simulink model "Copy_of_towing_project1"  (Simulink 10.1)
settings: Solver=ode4  StartTime=0.0  StopTime=200  FixedStep=1  RelTol=1e-3  EnableMultiTasking=on
PreLoadFcn:
  | load('Initialization_data.mat');
values from neighbouring files (symbols this model uses):
  D1 = [MM(1,1)/100, 0, 0; 0, MM(2,2)/40, 0; 0, 0, MM(3,3)/20]    [temp_code.m]
  M1 = diag([6.25e5, 6.25e5, 6.25e5*7.5^2])    [temp_code.m]
  Ma1 = [7.58e4, 0, 0; 0, 3.69e5 -1.4e5; 0, -1.4e5, 8.77e6]    [temp_code.m]
undefined symbols (not defined in the file or in its folder): magnitude
libraries: simulink_extras x4, simulink x4
settings Model: Creator=Lither  LastModifiedBy=Administrator
settings DataIOCC: LimitDataPoints=on
settings OptimizationCC: ExpressionDepthLimit=2147483647
settings DebuggingCC: FcnCallInpInsideContextMsg=warning  StateNameClashWarn=warning
settings ConfigComp: CovSFcnEnable=off

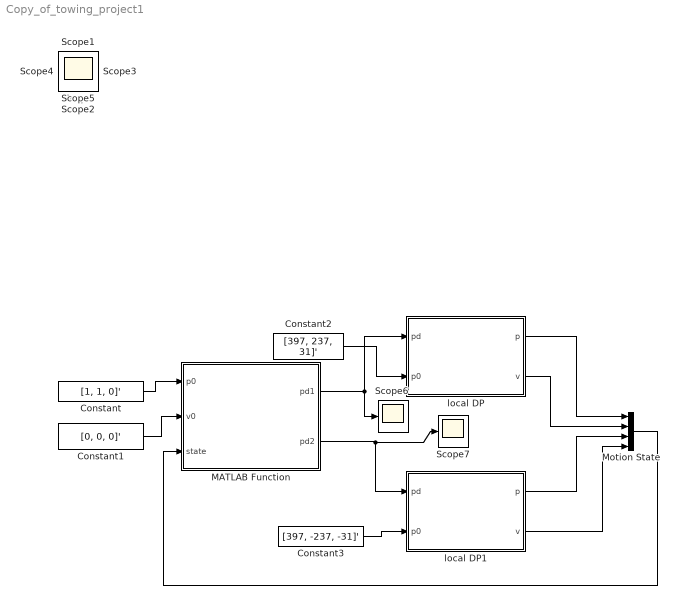
== system Copy_of_towing_project1 ==
  Constant : Constant  Value=[1, 1, 0]'
  Constant1 : Constant  Value=[0, 0, 0]'
  Constant2 : Constant  Value=[397, 237, 31]'
  Constant3 : Constant  Value=[397, -237, -31]'
  MATLAB Function : MATLAB Function  TreatAsAtomicUnit=on
  Motion State : Mux
  Scope{,1..7} (8 alike) : Scope
  local DP : Subsystem
  local DP1 : Subsystem
  wires:
  Constant/1 -> MATLAB Function/1(p0)
  Constant1/1 -> MATLAB Function/2(v0)
  MATLAB Function/1(pd1) -> local DP/1(pd), Scope6/1
  MATLAB Function/2(pd2) -> Scope7/1, local DP1/1(pd)
  Constant2/1 -> local DP/2(p0)
  Constant3/1 -> local DP1/2(p0)
  local DP/1(p) -> Motion State/1
  local DP/2(v) -> Motion State/2
  local DP1/1(p) -> Motion State/3
  local DP1/2(v) -> Motion State/4
  Motion State/1 -> MATLAB Function/3(state)

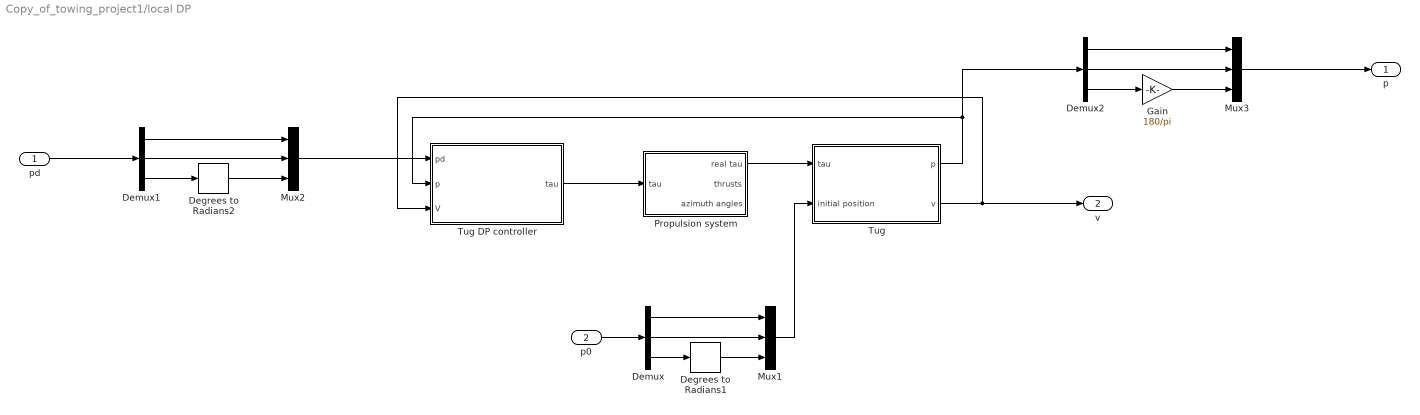
== system Copy_of_towing_project1/local DP ==
  pd : Inport
  p0 : Inport  Port=2
  Degrees to Radians1 : simulink_extras/Transformations/Degrees to Radians
  Degrees to Radians2 : simulink_extras/Transformations/Degrees to Radians
  Demux : Demux  Outputs=3
  Demux1 : Demux  Outputs=3
  Demux2 : Demux  Outputs=3
  Gain : Gain  Gain=180/pi
  Mux1 : Mux  Inputs=3
  Mux2 : Mux  Inputs=3
  Mux3 : Mux  Inputs=3
  Propulsion system : Subsystem  mask{f0=[1;1;1], a0=[50;60;70], u0=[1; 1; 1], wa=on}
      mask prompts: f0 "Initial values of thrusts"; a0 "Initial values of azimuth angles"; u0 "Thruster utilization"; wa "Show animation of thrust and azimuth angle"
  Tug : Subsystem  mask{wv=on}
      mask prompts: wv "Display animation of the vessel's motion"
  Tug DP controller : Subsystem  mask(Nonlinear DP Controller){Kp=diag([0.0028, 0.004, 0.0031]), Kd=diag([0.0573, 0.0716, 0.025]), Ki=diag([0.0028, 0.004, 0.0031])*0.01, WFF_gain=0}
      mask prompts: Kp "Proportional Gain Matrix: Kp"; Kd "Derivative Gain Matrix: Kd"; Ki "Integral Gain Matrix: Ki"; WFF_gain "Wave feedforward Gain"
      mask help: PID controller for Set-Point Reulation in Surge, Sway and Yaw
      mask Help:
      | The nonlinear  PID controller uses the rotation matrix in yaw for proper scaling of the surge, sway and yaw gains as a function of the yaw angle.
      | INPUTS: (1) eta_ref, (2) eta, (3) nu. OUPUTS: (1) tau.
      mask Display: disp('PID controller')
  p : Outport
  v : Outport  Port=2
  wires:
  Tug/2(v) -> v/1, Tug DP controller/3(V)
  Demux/2 -> Mux1/2
  Tug DP controller/1(tau) -> Propulsion system/1(tau)
  Demux1/2 -> Mux2/2
  Mux2/1 -> Tug DP controller/1(pd)
  Demux1/1 -> Mux2/1
  Degrees to Radians2/1 -> Mux2/3
  Demux1/3 -> Degrees to Radians2/1
  pd/1 -> Demux1/1
  Demux/1 -> Mux1/1
  Degrees to Radians1/1 -> Mux1/3
  Demux/3 -> Degrees to Radians1/1
  Propulsion system/1(real tau) -> Tug/1(tau)
  Mux1/1 -> Tug/2(initial position)
  p0/1 -> Demux/1
  Demux2/2 -> Mux3/2
  Tug/1(p) -> Demux2/1, Tug DP controller/2(p)
  Mux3/1 -> p/1
  Demux2/3 -> Gain/1
  Gain/1 -> Mux3/3
  Demux2/1 -> Mux3/1

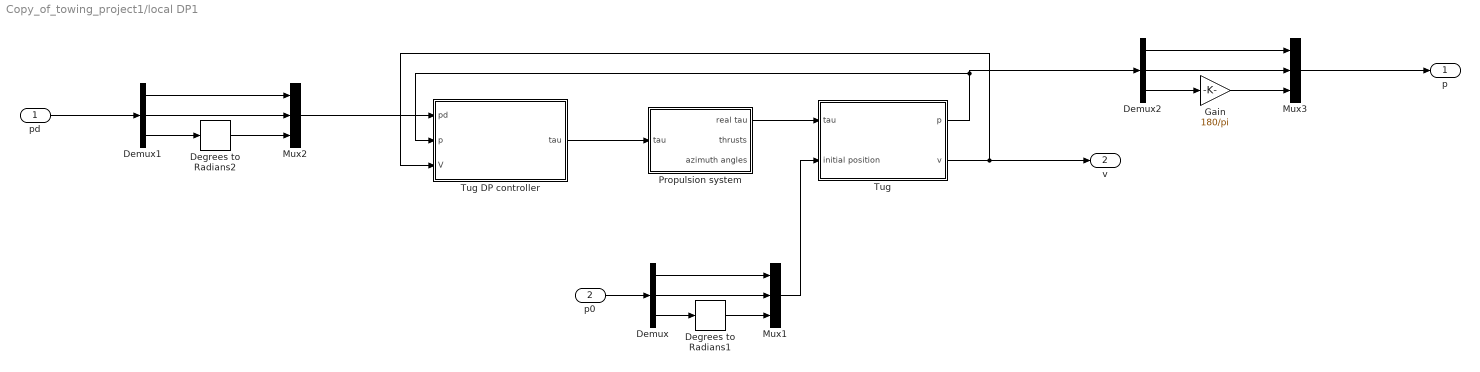
== system Copy_of_towing_project1/local DP1 ==
  pd : Inport
  p0 : Inport  Port=2
  Degrees to Radians1 : simulink_extras/Transformations/Degrees to Radians
  Degrees to Radians2 : simulink_extras/Transformations/Degrees to Radians
  Demux : Demux  Outputs=3
  Demux1 : Demux  Outputs=3
  Demux2 : Demux  Outputs=3
  Gain : Gain  Gain=180/pi
  Mux1 : Mux  Inputs=3
  Mux2 : Mux  Inputs=3
  Mux3 : Mux  Inputs=3
  Propulsion system : Subsystem  mask{f0=[1;1;1], a0=[50;60;70], u0=[1; 1; 1], wa=on}
      mask prompts: f0 "Initial values of thrusts"; a0 "Initial values of azimuth angles"; u0 "Thruster utilization"; wa "Show animation of thrust and azimuth angle"
  Tug : Subsystem  mask{wv=on}
      mask prompts: wv "Display animation of the vessel's motion"
  Tug DP controller : Subsystem  mask(Nonlinear DP Controller){Kp=diag([0.0028, 0.004, 0.0031]), Kd=diag([0.0573, 0.0716, 0.025]), Ki=diag([0.0028, 0.004, 0.0031])*0.01, WFF_gain=0}
      mask prompts: Kp "Proportional Gain Matrix: Kp"; Kd "Derivative Gain Matrix: Kd"; Ki "Integral Gain Matrix: Ki"; WFF_gain "Wave feedforward Gain"
      mask help: PID controller for Set-Point Reulation in Surge, Sway and Yaw
      mask Help:
      | The nonlinear  PID controller uses the rotation matrix in yaw for proper scaling of the surge, sway and yaw gains as a function of the yaw angle.
      | INPUTS: (1) eta_ref, (2) eta, (3) nu. OUPUTS: (1) tau.
      mask Display: disp('PID controller')
  p : Outport
  v : Outport  Port=2
  wires:
  Tug/2(v) -> v/1, Tug DP controller/3(V)
  Demux/2 -> Mux1/2
  Tug DP controller/1(tau) -> Propulsion system/1(tau)
  Demux1/2 -> Mux2/2
  Mux2/1 -> Tug DP controller/1(pd)
  Demux1/1 -> Mux2/1
  Degrees to Radians2/1 -> Mux2/3
  Demux1/3 -> Degrees to Radians2/1
  pd/1 -> Demux1/1
  Demux/1 -> Mux1/1
  Degrees to Radians1/1 -> Mux1/3
  Demux/3 -> Degrees to Radians1/1
  Propulsion system/1(real tau) -> Tug/1(tau)
  Mux1/1 -> Tug/2(initial position)
  p0/1 -> Demux/1
  Mux3/1 -> p/1
  Tug/1(p) -> Demux2/1, Tug DP controller/2(p)
  Demux2/3 -> Gain/1
  Demux2/2 -> Mux3/2
  Gain/1 -> Mux3/3
  Demux2/1 -> Mux3/1

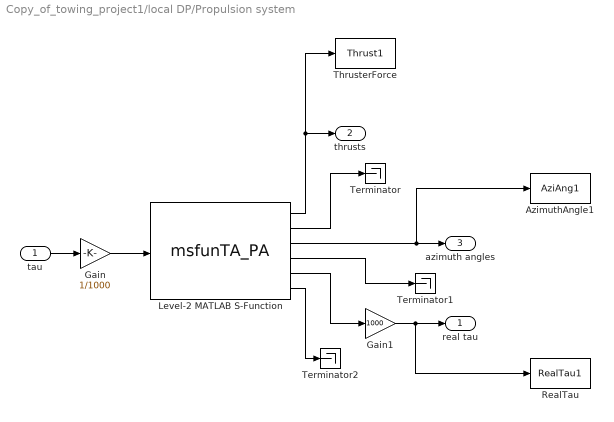
== system Copy_of_towing_project1/local DP/Propulsion system ==
  tau : Inport
  AzimuthAngle1 : ToWorkspace  VariableName=AziAng1  SampleTime=-1
  Gain : Gain  Gain=1/1000
  Gain1 : Gain  Gain=1000
  Level-2 MATLAB S-Function : M-S-Function  FunctionName=msfunTA_PA  Parameters=f0,a0,wa
  RealTau : ToWorkspace  VariableName=RealTau1  SampleTime=-1
  Terminator : Terminator
  Terminator1 : Terminator
  Terminator2 : Terminator
  ThrusterForce : ToWorkspace  VariableName=Thrust1  SampleTime=-1
  real tau : Outport
  thrusts : Outport  Port=2
  azimuth angles : Outport  Port=3
  wires:
  tau/1 -> Gain/1
  Level-2 MATLAB S-Function/2 -> Terminator/1
  Level-2 MATLAB S-Function/3 -> AzimuthAngle1/1, azimuth angles/1
  Level-2 MATLAB S-Function/4 -> Terminator1/1
  Level-2 MATLAB S-Function/5 -> Gain1/1
  Level-2 MATLAB S-Function/6 -> Terminator2/1
  Level-2 MATLAB S-Function/1 -> ThrusterForce/1, thrusts/1
  Gain/1 -> Level-2 MATLAB S-Function/1
  Gain1/1 -> RealTau/1, real tau/1

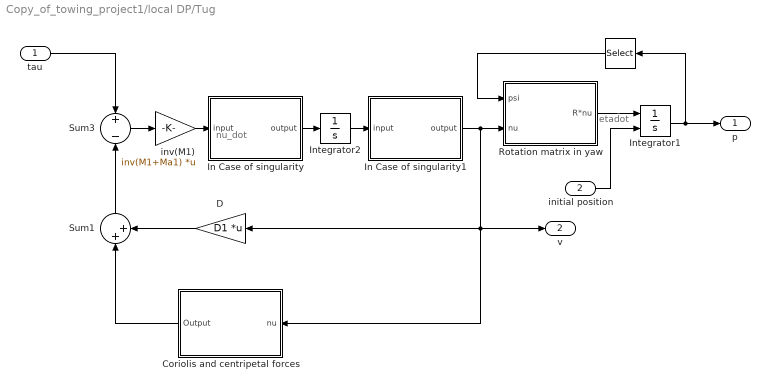
== system Copy_of_towing_project1/local DP/Tug ==
  note: nu_dot
  note: etadot
  tau : Inport
  initial position : Inport  Port=2
  " " : Selector  InputPortWidth=3  IndexOptions=Index vector (dialog)  Indices=[3]  OutputSizes=1
  Coriolis and centripetal forces : Subsystem
  D : Gain  Gain=D1  Multiplication=Matrix(K*u)  SaturateOnIntegerOverflow=on  OutDataTypeStr=Inherit: Same as input  ParamDataTypeStr=Inherit: Same as input
  In Case of singularity : Subsystem
  In Case of singularity1 : Subsystem
  Integrator1 : Integrator  InitialConditionSource=external  InitialCondition=1.05
  Integrator2 : Integrator
  Rotation matrix in yaw : Subsystem
  Sum1 : Sum  Inputs=|++  InputSameDT=on  SaturateOnIntegerOverflow=on  OutDataTypeStr=Inherit: Same as first input
  Sum3 : Sum  Inputs=+-  InputSameDT=on  SaturateOnIntegerOverflow=on  OutDataTypeStr=Inherit: Same as first input
  inv(M1) : Gain  Gain=inv(M1+Ma1)  Multiplication=Matrix(K*u)  SaturateOnIntegerOverflow=on  OutDataTypeStr=Inherit: Same as input  ParamDataTypeStr=Inherit: Same as input
  p : Outport
  v : Outport  Port=2
  wires:
  Sum3/1 -> inv(M1)/1
  inv(M1)/1 -> In Case of singularity/1(input)
  Rotation matrix in yaw/1(R*nu) -> Integrator1/1
  Integrator1/1 -> p/1, " "/1
  " "/1 -> Rotation matrix in yaw/1(psi)
  tau/1 -> Sum3/1
  initial position/1 -> Integrator1/2
  Integrator2/1 -> In Case of singularity1/1(input)
  In Case of singularity/1(output) -> Integrator2/1
  In Case of singularity1/1(output) -> Rotation matrix in yaw/2(nu), D/1, Coriolis and centripetal forces/1(nu), v/1
  D/1 -> Sum1/2
  Coriolis and centripetal forces/1(Output) -> Sum1/1
  Sum1/1 -> Sum3/2

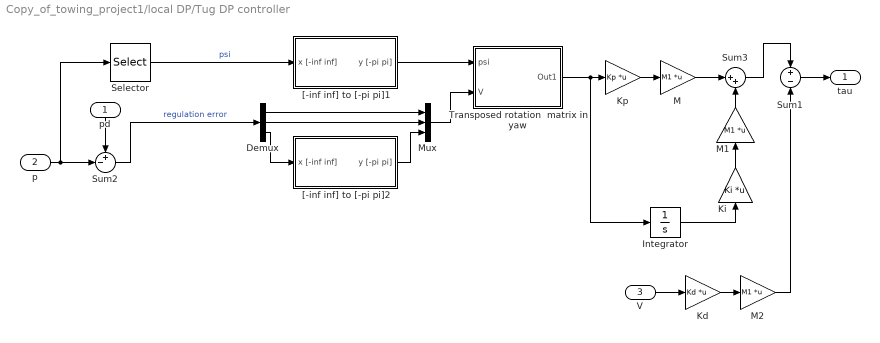
== system Copy_of_towing_project1/local DP/Tug DP controller ==
  pd : Inport
  p : Inport  Port=2
  V : Inport  Port=3
  Demux : Demux  Outputs=3
  Integrator : Integrator
  Kd : Gain  Gain=Kd  Multiplication=Matrix(K*u)  SaturateOnIntegerOverflow=on  OutDataTypeStr=Inherit: Same as input  ParamDataTypeStr=Inherit: Same as input
  Ki : Gain  Gain=Ki  Multiplication=Matrix(K*u)  SaturateOnIntegerOverflow=on  OutDataTypeStr=Inherit: Same as input  ParamDataTypeStr=Inherit: Same as input
  Kp : Gain  Gain=Kp  Multiplication=Matrix(K*u)  SaturateOnIntegerOverflow=on  OutDataTypeStr=Inherit: Same as input  ParamDataTypeStr=Inherit: Same as input
  M : Gain  Gain=M1  Multiplication=Matrix(K*u)  SaturateOnIntegerOverflow=on  OutDataTypeStr=Inherit: Same as input  ParamDataTypeStr=Inherit: Same as input
  M1 : Gain  Gain=M1  Multiplication=Matrix(K*u)  SaturateOnIntegerOverflow=on  OutDataTypeStr=Inherit: Same as input  ParamDataTypeStr=Inherit: Same as input
  M2 : Gain  Gain=M1  Multiplication=Matrix(K*u)  SaturateOnIntegerOverflow=on  OutDataTypeStr=Inherit: Same as input  ParamDataTypeStr=Inherit: Same as input
  Mux : Mux  Inputs=3
  Selector : Selector  InputPortWidth=3  IndexOptions=Index vector (dialog)  Indices=[ 3]  OutputSizes=1
  Sum1 : Sum  Inputs=+-  InputSameDT=on  SaturateOnIntegerOverflow=on  OutDataTypeStr=Inherit: Same as first input
  Sum2 : Sum  Inputs=+-|  InputSameDT=on  SaturateOnIntegerOverflow=on  OutDataTypeStr=Inherit: Same as first input
  Sum3 : Sum  Inputs=|++  InputSameDT=on  SaturateOnIntegerOverflow=on  OutDataTypeStr=Inherit: Same as first input
  Transposed rotation  matrix in yaw : Subsystem
  "[-inf inf] to [-pi pi]1" : Subsystem
  "[-inf inf] to [-pi pi]2" : Subsystem
  tau : Outport  InitialOutput=0
  wires:
  "[-inf inf] to [-pi pi]1"/1(y [-pi pi]) -> Transposed rotation  matrix in yaw/1(psi)
  Selector/1 -> "[-inf inf] to [-pi pi]1"/1(x [-inf inf])  "psi"
  Mux/1 -> Transposed rotation  matrix in yaw/2(V)
  Demux/1 -> Mux/1
  Demux/2 -> Mux/2
  "[-inf inf] to [-pi pi]2"/1(y [-pi pi]) -> Mux/3
  Sum2/1 -> Demux/1  "regulation error"
  Demux/3 -> "[-inf inf] to [-pi pi]2"/1(x [-inf inf])
  pd/1 -> Sum2/1
  Sum1/1 -> tau/1
  p/1 -> Sum2/2, Selector/1
  V/1 -> Kd/1
  Integrator/1 -> Ki/1
  Kp/1 -> M/1
  Ki/1 -> M1/1
  Transposed rotation  matrix in yaw/1(Out1) -> Kp/1, Integrator/1
  Kd/1 -> M2/1
  M/1 -> Sum3/1
  M1/1 -> Sum3/2
  Sum3/1 -> Sum1/1
  M2/1 -> Sum1/2

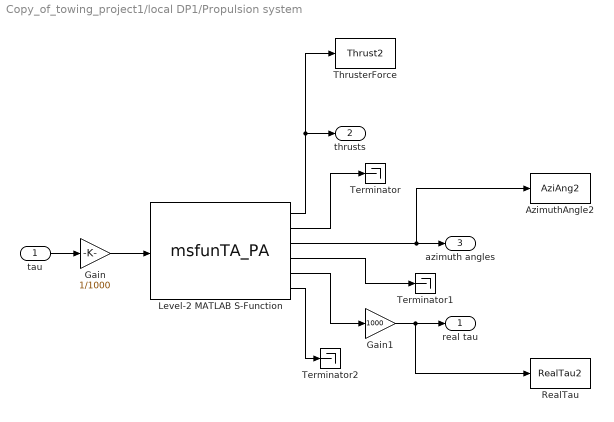
== system Copy_of_towing_project1/local DP1/Propulsion system ==
  tau : Inport
  AzimuthAngle2 : ToWorkspace  VariableName=AziAng2  SampleTime=-1
  Gain : Gain  Gain=1/1000
  Gain1 : Gain  Gain=1000
  Level-2 MATLAB S-Function : M-S-Function  FunctionName=msfunTA_PA  Parameters=f0,a0,wa
  RealTau : ToWorkspace  VariableName=RealTau2  SampleTime=-1
  Terminator : Terminator
  Terminator1 : Terminator
  Terminator2 : Terminator
  ThrusterForce : ToWorkspace  VariableName=Thrust2  SampleTime=-1
  real tau : Outport
  thrusts : Outport  Port=2
  azimuth angles : Outport  Port=3
  wires:
  tau/1 -> Gain/1
  Level-2 MATLAB S-Function/2 -> Terminator/1
  Level-2 MATLAB S-Function/3 -> AzimuthAngle2/1, azimuth angles/1
  Level-2 MATLAB S-Function/4 -> Terminator1/1
  Level-2 MATLAB S-Function/5 -> Gain1/1
  Level-2 MATLAB S-Function/6 -> Terminator2/1
  Level-2 MATLAB S-Function/1 -> ThrusterForce/1, thrusts/1
  Gain/1 -> Level-2 MATLAB S-Function/1
  Gain1/1 -> RealTau/1, real tau/1

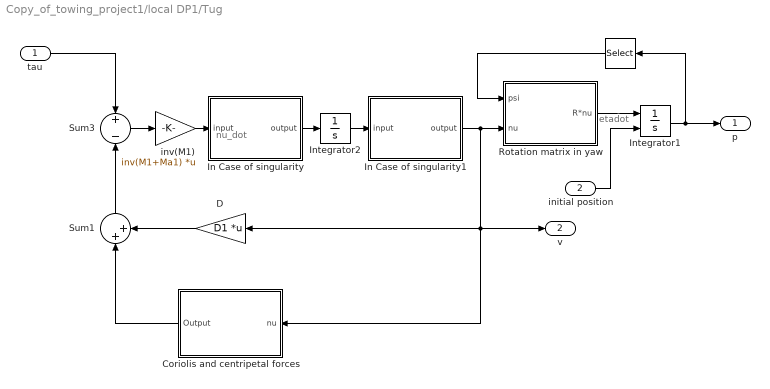
== system Copy_of_towing_project1/local DP1/Tug ==
  note: nu_dot
  note: etadot
  tau : Inport
  initial position : Inport  Port=2
  " " : Selector  InputPortWidth=3  IndexOptions=Index vector (dialog)  Indices=[3]  OutputSizes=1
  Coriolis and centripetal forces : Subsystem
  D : Gain  Gain=D1  Multiplication=Matrix(K*u)  SaturateOnIntegerOverflow=on  OutDataTypeStr=Inherit: Same as input  ParamDataTypeStr=Inherit: Same as input
  In Case of singularity : Subsystem
  In Case of singularity1 : Subsystem
  Integrator1 : Integrator  InitialConditionSource=external  InitialCondition=1.05
  Integrator2 : Integrator
  Rotation matrix in yaw : Subsystem
  Sum1 : Sum  Inputs=|++  InputSameDT=on  SaturateOnIntegerOverflow=on  OutDataTypeStr=Inherit: Same as first input
  Sum3 : Sum  Inputs=+-  InputSameDT=on  SaturateOnIntegerOverflow=on  OutDataTypeStr=Inherit: Same as first input
  inv(M1) : Gain  Gain=inv(M1+Ma1)  Multiplication=Matrix(K*u)  SaturateOnIntegerOverflow=on  OutDataTypeStr=Inherit: Same as input  ParamDataTypeStr=Inherit: Same as input
  p : Outport
  v : Outport  Port=2
  wires:
  Sum3/1 -> inv(M1)/1
  inv(M1)/1 -> In Case of singularity/1(input)
  Rotation matrix in yaw/1(R*nu) -> Integrator1/1
  Integrator1/1 -> p/1, " "/1
  " "/1 -> Rotation matrix in yaw/1(psi)
  tau/1 -> Sum3/1
  initial position/1 -> Integrator1/2
  Integrator2/1 -> In Case of singularity1/1(input)
  In Case of singularity/1(output) -> Integrator2/1
  In Case of singularity1/1(output) -> Rotation matrix in yaw/2(nu), D/1, Coriolis and centripetal forces/1(nu), v/1
  D/1 -> Sum1/2
  Coriolis and centripetal forces/1(Output) -> Sum1/1
  Sum1/1 -> Sum3/2

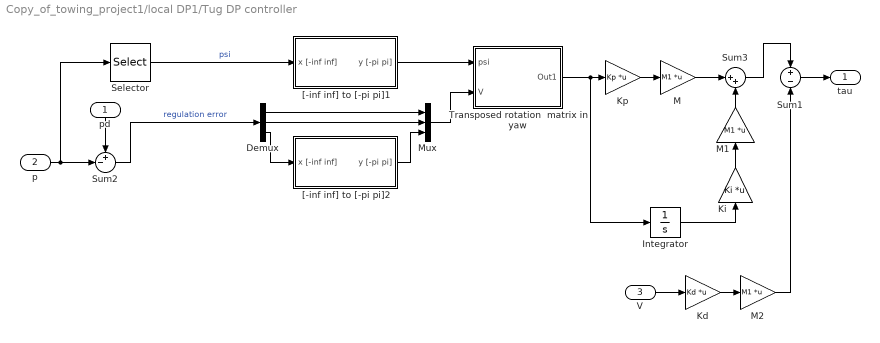
== system Copy_of_towing_project1/local DP1/Tug DP controller ==
  pd : Inport
  p : Inport  Port=2
  V : Inport  Port=3
  Demux : Demux  Outputs=3
  Integrator : Integrator
  Kd : Gain  Gain=Kd  Multiplication=Matrix(K*u)  SaturateOnIntegerOverflow=on  OutDataTypeStr=Inherit: Same as input  ParamDataTypeStr=Inherit: Same as input
  Ki : Gain  Gain=Ki  Multiplication=Matrix(K*u)  SaturateOnIntegerOverflow=on  OutDataTypeStr=Inherit: Same as input  ParamDataTypeStr=Inherit: Same as input
  Kp : Gain  Gain=Kp  Multiplication=Matrix(K*u)  SaturateOnIntegerOverflow=on  OutDataTypeStr=Inherit: Same as input  ParamDataTypeStr=Inherit: Same as input
  M : Gain  Gain=M1  Multiplication=Matrix(K*u)  SaturateOnIntegerOverflow=on  OutDataTypeStr=Inherit: Same as input  ParamDataTypeStr=Inherit: Same as input
  M1 : Gain  Gain=M1  Multiplication=Matrix(K*u)  SaturateOnIntegerOverflow=on  OutDataTypeStr=Inherit: Same as input  ParamDataTypeStr=Inherit: Same as input
  M2 : Gain  Gain=M1  Multiplication=Matrix(K*u)  SaturateOnIntegerOverflow=on  OutDataTypeStr=Inherit: Same as input  ParamDataTypeStr=Inherit: Same as input
  Mux : Mux  Inputs=3
  Selector : Selector  InputPortWidth=3  IndexOptions=Index vector (dialog)  Indices=[ 3]  OutputSizes=1
  Sum1 : Sum  Inputs=+-  InputSameDT=on  SaturateOnIntegerOverflow=on  OutDataTypeStr=Inherit: Same as first input
  Sum2 : Sum  Inputs=+-|  InputSameDT=on  SaturateOnIntegerOverflow=on  OutDataTypeStr=Inherit: Same as first input
  Sum3 : Sum  Inputs=|++  InputSameDT=on  SaturateOnIntegerOverflow=on  OutDataTypeStr=Inherit: Same as first input
  Transposed rotation  matrix in yaw : Subsystem
  "[-inf inf] to [-pi pi]1" : Subsystem
  "[-inf inf] to [-pi pi]2" : Subsystem
  tau : Outport  InitialOutput=0
  wires:
  "[-inf inf] to [-pi pi]1"/1(y [-pi pi]) -> Transposed rotation  matrix in yaw/1(psi)
  Selector/1 -> "[-inf inf] to [-pi pi]1"/1(x [-inf inf])  "psi"
  Mux/1 -> Transposed rotation  matrix in yaw/2(V)
  Demux/1 -> Mux/1
  Demux/2 -> Mux/2
  "[-inf inf] to [-pi pi]2"/1(y [-pi pi]) -> Mux/3
  Sum2/1 -> Demux/1  "regulation error"
  Demux/3 -> "[-inf inf] to [-pi pi]2"/1(x [-inf inf])
  pd/1 -> Sum2/1
  Sum1/1 -> tau/1
  p/1 -> Sum2/2, Selector/1
  V/1 -> Kd/1
  Integrator/1 -> Ki/1
  Kp/1 -> M/1
  Ki/1 -> M1/1
  Transposed rotation  matrix in yaw/1(Out1) -> Kp/1, Integrator/1
  Kd/1 -> M2/1
  M/1 -> Sum3/1
  M1/1 -> Sum3/2
  Sum3/1 -> Sum1/1
  M2/1 -> Sum1/2

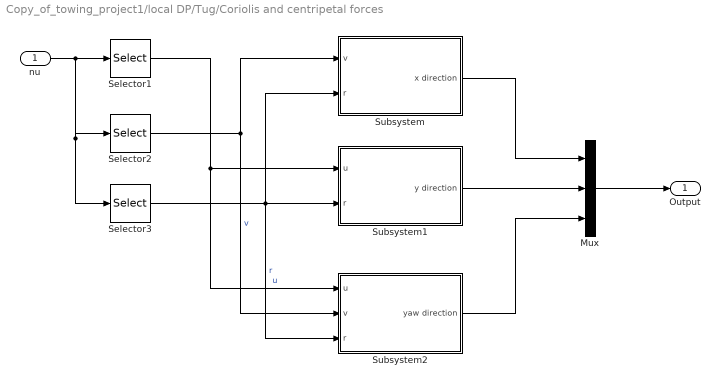
== system Copy_of_towing_project1/local DP/Tug/Coriolis and centripetal forces ==
  nu : Inport
  Mux : Mux  Inputs=3
  Selector1 : Selector  InputPortWidth=3  IndexOptions=Index vector (dialog)  Indices=[1 ]  OutputSizes=1
  Selector2 : Selector  InputPortWidth=3  IndexOptions=Index vector (dialog)  Indices=[2]  OutputSizes=1
  Selector3 : Selector  InputPortWidth=3  IndexOptions=Index vector (dialog)  Indices=[3]  OutputSizes=1
  Subsystem : Subsystem
  Subsystem1 : Subsystem
  Subsystem2 : Subsystem
  Output : Outport
  wires:
  nu/1 -> Selector1/1, Selector2/1, Selector3/1
  Selector2/1 -> Subsystem/1(v), Subsystem2/2(v)  "v"
  Selector3/1 -> Subsystem/2(r), Subsystem1/2(r), Subsystem2/3(r)  "r"
  Selector1/1 -> Subsystem1/1(u), Subsystem2/1(u)  "u"
  Subsystem/1(x direction) -> Mux/1
  Subsystem1/1(y direction) -> Mux/2
  Subsystem2/1(yaw direction) -> Mux/3
  Mux/1 -> Output/1

== system Copy_of_towing_project1/local DP/Tug/In Case of singularity ==
  input : Inport
  Compare To Constant : simulink/Logic and Bit Operations/Compare To Constant  relop=>=  const=1e8  OutDataTypeStr=boolean
  Stop Simulation : Stop
  output : Outport
  wires:
  input/1 -> output/1, Compare To Constant/1
  Compare To Constant/1 -> Stop Simulation/1

== system Copy_of_towing_project1/local DP/Tug/In Case of singularity1 ==
  input : Inport
  Compare To Constant : simulink/Logic and Bit Operations/Compare To Constant  relop=>=  const=1e10  OutDataTypeStr=boolean
  Stop Simulation : Stop
  output : Outport
  wires:
  input/1 -> output/1, Compare To Constant/1
  Compare To Constant/1 -> Stop Simulation/1

== system Copy_of_towing_project1/local DP/Tug/Rotation matrix in yaw ==
  psi : Inport
  nu : Inport  Port=2
  Fcn : Fcn  Expr=cos(u(1))*u(2)-sin(u(1))*u(3)
  Fcn1 : Fcn  Expr=sin(u(1))*u(2)+cos(u(1))*u(3)
  Fcn2 : Fcn  Expr=u(4)
  Mux : Mux  Inputs=2
  Mux1 : Mux  Inputs=3
  R*nu : Outport
  wires:
  Mux1/1 -> R*nu/1  "eta_dot"
  Mux/1 -> Fcn/1, Fcn1/1, Fcn2/1
  psi/1 -> Mux/1
  nu/1 -> Mux/2
  Fcn1/1 -> Mux1/2  "y_dot"
  Fcn/1 -> Mux1/1  "x_dot"
  Fcn2/1 -> Mux1/3  "psi_dot"

== system Copy_of_towing_project1/local DP/Tug DP controller/Transposed rotation  matrix in yaw ==
  psi : Inport
  V : Inport  Port=2
  Mux : Mux  Inputs=2
  Mux1 : Mux  Inputs=3
  Row1 : Fcn  Expr=cos(u(1))*u(2)+sin(u(1))*u(3)
  Row2 : Fcn  Expr=-sin(u(1))*u(2)+cos(u(1))*u(3)
  Row3 : Fcn  Expr=u(4)
  Out1 : Outport
  wires:
  Mux/1 -> Row3/1, Row2/1, Row1/1
  Row1/1 -> Mux1/1
  Row2/1 -> Mux1/2
  Row3/1 -> Mux1/3
  Mux1/1 -> Out1/1
  psi/1 -> Mux/1
  V/1 -> Mux/2

== system Copy_of_towing_project1/local DP/Tug DP controller/[-inf inf] to [-pi pi]1 ==
  note: x
  note: r
  x [-inf inf] : Inport
  Constant : Constant  Value=2*pi
  Gain : Gain  Gain=pi  SaturateOnIntegerOverflow=on  OutDataTypeStr=Inherit: Same as input  ParamDataTypeStr=Inherit: Same as input
  Math Function : Math  Operator=rem  SignedPower=on  SaturateOnIntegerOverflow=on
  Saturation : Saturate  UpperLimit=1e10  LowerLimit=-1e10
  Sign : Signum
  Sum : Sum  Inputs=|+-  SaturateOnIntegerOverflow=on
  Sum1 : Sum  Inputs=|++  SaturateOnIntegerOverflow=on
  y [-pi pi] : Outport
  wires:
  x [-inf inf]/1 -> Saturation/1
  Sign/1 -> Gain/1
  Gain/1 -> Sum/2, Sum1/2
  Sum1/1 -> Math Function/1
  Constant/1 -> Math Function/2
  Math Function/1 -> Sum/1
  Sum/1 -> y [-pi pi]/1
  Saturation/1 -> Sum1/1, Sign/1

== system Copy_of_towing_project1/local DP/Tug DP controller/[-inf inf] to [-pi pi]2 ==
  note: r
  note: x
  x [-inf inf] : Inport
  Constant : Constant  Value=2*pi
  Gain : Gain  Gain=pi  SaturateOnIntegerOverflow=on  OutDataTypeStr=Inherit: Same as input  ParamDataTypeStr=Inherit: Same as input
  Math Function : Math  Operator=rem  SignedPower=on  SaturateOnIntegerOverflow=on
  Saturation : Saturate  UpperLimit=1e10  LowerLimit=-1e10
  Sign : Signum
  Sum : Sum  Inputs=|+-  SaturateOnIntegerOverflow=on
  Sum1 : Sum  Inputs=|++  SaturateOnIntegerOverflow=on
  y [-pi pi] : Outport
  wires:
  Saturation/1 -> Sign/1, Sum1/1
  Sum/1 -> y [-pi pi]/1
  Math Function/1 -> Sum/1
  Constant/1 -> Math Function/2
  Sum1/1 -> Math Function/1
  Gain/1 -> Sum1/2, Sum/2
  Sign/1 -> Gain/1
  x [-inf inf]/1 -> Saturation/1

== system Copy_of_towing_project1/local DP1/Tug/Coriolis and centripetal forces ==
  nu : Inport
  Mux : Mux  Inputs=3
  Selector1 : Selector  InputPortWidth=3  IndexOptions=Index vector (dialog)  Indices=[1 ]  OutputSizes=1
  Selector2 : Selector  InputPortWidth=3  IndexOptions=Index vector (dialog)  Indices=[2]  OutputSizes=1
  Selector3 : Selector  InputPortWidth=3  IndexOptions=Index vector (dialog)  Indices=[3]  OutputSizes=1
  Subsystem : Subsystem
  Subsystem1 : Subsystem
  Subsystem2 : Subsystem
  Output : Outport
  wires:
  nu/1 -> Selector1/1, Selector2/1, Selector3/1
  Selector2/1 -> Subsystem/1(v), Subsystem2/2(v)  "v"
  Selector3/1 -> Subsystem/2(r), Subsystem1/2(r), Subsystem2/3(r)  "r"
  Selector1/1 -> Subsystem1/1(u), Subsystem2/1(u)  "u"
  Subsystem/1(x direction) -> Mux/1
  Subsystem1/1(y direction) -> Mux/2
  Subsystem2/1(yaw direction) -> Mux/3
  Mux/1 -> Output/1

== system Copy_of_towing_project1/local DP1/Tug/In Case of singularity ==
  input : Inport
  Compare To Constant : simulink/Logic and Bit Operations/Compare To Constant  relop=>=  const=1e8  OutDataTypeStr=boolean
  Stop Simulation : Stop
  output : Outport
  wires:
  input/1 -> output/1, Compare To Constant/1
  Compare To Constant/1 -> Stop Simulation/1

== system Copy_of_towing_project1/local DP1/Tug/In Case of singularity1 ==
  input : Inport
  Compare To Constant : simulink/Logic and Bit Operations/Compare To Constant  relop=>=  const=1e10  OutDataTypeStr=boolean
  Stop Simulation : Stop
  output : Outport
  wires:
  input/1 -> output/1, Compare To Constant/1
  Compare To Constant/1 -> Stop Simulation/1

== system Copy_of_towing_project1/local DP1/Tug/Rotation matrix in yaw ==
  psi : Inport
  nu : Inport  Port=2
  Fcn : Fcn  Expr=cos(u(1))*u(2)-sin(u(1))*u(3)
  Fcn1 : Fcn  Expr=sin(u(1))*u(2)+cos(u(1))*u(3)
  Fcn2 : Fcn  Expr=u(4)
  Mux : Mux  Inputs=2
  Mux1 : Mux  Inputs=3
  R*nu : Outport
  wires:
  Mux1/1 -> R*nu/1  "eta_dot"
  Mux/1 -> Fcn/1, Fcn1/1, Fcn2/1
  psi/1 -> Mux/1
  nu/1 -> Mux/2
  Fcn1/1 -> Mux1/2  "y_dot"
  Fcn/1 -> Mux1/1  "x_dot"
  Fcn2/1 -> Mux1/3  "psi_dot"

== system Copy_of_towing_project1/local DP1/Tug DP controller/Transposed rotation  matrix in yaw ==
  psi : Inport
  V : Inport  Port=2
  Mux : Mux  Inputs=2
  Mux1 : Mux  Inputs=3
  Row1 : Fcn  Expr=cos(u(1))*u(2)+sin(u(1))*u(3)
  Row2 : Fcn  Expr=-sin(u(1))*u(2)+cos(u(1))*u(3)
  Row3 : Fcn  Expr=u(4)
  Out1 : Outport
  wires:
  Mux/1 -> Row3/1, Row2/1, Row1/1
  Row1/1 -> Mux1/1
  Row2/1 -> Mux1/2
  Row3/1 -> Mux1/3
  Mux1/1 -> Out1/1
  psi/1 -> Mux/1
  V/1 -> Mux/2

== system Copy_of_towing_project1/local DP1/Tug DP controller/[-inf inf] to [-pi pi]1 ==
  note: x
  note: r
  x [-inf inf] : Inport
  Constant : Constant  Value=2*pi
  Gain : Gain  Gain=pi  SaturateOnIntegerOverflow=on  OutDataTypeStr=Inherit: Same as input  ParamDataTypeStr=Inherit: Same as input
  Math Function : Math  Operator=rem  SignedPower=on  SaturateOnIntegerOverflow=on
  Saturation : Saturate  UpperLimit=1e10  LowerLimit=-1e10
  Sign : Signum
  Sum : Sum  Inputs=|+-  SaturateOnIntegerOverflow=on
  Sum1 : Sum  Inputs=|++  SaturateOnIntegerOverflow=on
  y [-pi pi] : Outport
  wires:
  x [-inf inf]/1 -> Saturation/1
  Sign/1 -> Gain/1
  Gain/1 -> Sum/2, Sum1/2
  Sum1/1 -> Math Function/1
  Constant/1 -> Math Function/2
  Math Function/1 -> Sum/1
  Sum/1 -> y [-pi pi]/1
  Saturation/1 -> Sum1/1, Sign/1

== system Copy_of_towing_project1/local DP1/Tug DP controller/[-inf inf] to [-pi pi]2 ==
  note: r
  note: x
  x [-inf inf] : Inport
  Constant : Constant  Value=2*pi
  Gain : Gain  Gain=pi  SaturateOnIntegerOverflow=on  OutDataTypeStr=Inherit: Same as input  ParamDataTypeStr=Inherit: Same as input
  Math Function : Math  Operator=rem  SignedPower=on  SaturateOnIntegerOverflow=on
  Saturation : Saturate  UpperLimit=1e10  LowerLimit=-1e10
  Sign : Signum
  Sum : Sum  Inputs=|+-  SaturateOnIntegerOverflow=on
  Sum1 : Sum  Inputs=|++  SaturateOnIntegerOverflow=on
  y [-pi pi] : Outport
  wires:
  Saturation/1 -> Sign/1, Sum1/1
  Sum/1 -> y [-pi pi]/1
  Math Function/1 -> Sum/1
  Constant/1 -> Math Function/2
  Sum1/1 -> Math Function/1
  Gain/1 -> Sum1/2, Sum/2
  Sign/1 -> Gain/1
  x [-inf inf]/1 -> Saturation/1

== system Copy_of_towing_project1/local DP/Tug/Coriolis and centripetal forces/Subsystem ==
  v : Inport
  r : Inport  Port=2
  -a22 : Gain  Gain=-M1(2,2)-Ma1(2,2)  Multiplication=Matrix(K*u)  SaturateOnIntegerOverflow=on  OutDataTypeStr=Inherit: Same as input  ParamDataTypeStr=Inherit: Same as input
  -a26 : Gain  Gain=-M1(2,3)-Ma1(2,3)  Multiplication=Matrix(K*u)  SaturateOnIntegerOverflow=on  OutDataTypeStr=Inherit: Same as input  ParamDataTypeStr=Inherit: Same as input
  Add : Sum
  Math Function : Math  Operator=magnitude^2  SignedPower=on  SaturateOnIntegerOverflow=on
  Product : Product  RndMeth=Zero
  x direction : Outport
  wires:
  v/1 -> Product/1
  r/1 -> Product/2, Math Function/1
  Product/1 -> -a22/1
  Math Function/1 -> -a26/1
  -a22/1 -> Add/1
  -a26/1 -> Add/2
  Add/1 -> x direction/1

== system Copy_of_towing_project1/local DP/Tug/Coriolis and centripetal forces/Subsystem1 ==
  u : Inport
  r : Inport  Port=2
  Product : Product  RndMeth=Zero
  a11 : Gain  Gain=M1(1,1)+Ma1(1,1)  Multiplication=Matrix(K*u)  SaturateOnIntegerOverflow=on  OutDataTypeStr=Inherit: Same as input  ParamDataTypeStr=Inherit: Same as input
  y direction : Outport
  wires:
  Product/1 -> a11/1
  r/1 -> Product/2
  u/1 -> Product/1
  a11/1 -> y direction/1

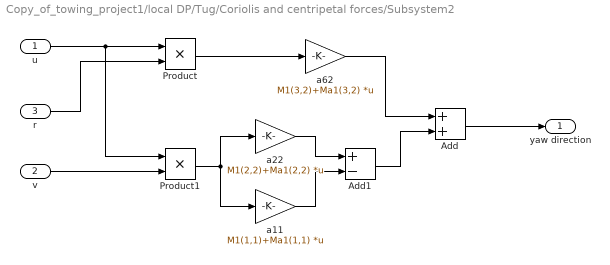
== system Copy_of_towing_project1/local DP/Tug/Coriolis and centripetal forces/Subsystem2 ==
  u : Inport
  v : Inport  Port=2
  r : Inport  Port=3
  Add : Sum
  Add1 : Sum  Inputs=+-
  Product : Product  RndMeth=Zero
  Product1 : Product  RndMeth=Zero
  a11 : Gain  Gain=M1(1,1)+Ma1(1,1)  Multiplication=Matrix(K*u)  SaturateOnIntegerOverflow=on  OutDataTypeStr=Inherit: Same as input  ParamDataTypeStr=Inherit: Same as input
  a22 : Gain  Gain=M1(2,2)+Ma1(2,2)  Multiplication=Matrix(K*u)  SaturateOnIntegerOverflow=on  OutDataTypeStr=Inherit: Same as input  ParamDataTypeStr=Inherit: Same as input
  a62 : Gain  Gain=M1(3,2)+Ma1(3,2)  Multiplication=Matrix(K*u)  SaturateOnIntegerOverflow=on  OutDataTypeStr=Inherit: Same as input  ParamDataTypeStr=Inherit: Same as input
  yaw direction : Outport
  wires:
  u/1 -> Product/1, Product1/1
  r/1 -> Product/2
  Product/1 -> a62/1
  v/1 -> Product1/2
  Product1/1 -> a22/1, a11/1
  a22/1 -> Add1/1
  a11/1 -> Add1/2
  Add1/1 -> Add/2
  a62/1 -> Add/1
  Add/1 -> yaw direction/1

== system Copy_of_towing_project1/local DP1/Tug/Coriolis and centripetal forces/Subsystem ==
  v : Inport
  r : Inport  Port=2
  -a22 : Gain  Gain=-M1(2,2)-Ma1(2,2)  Multiplication=Matrix(K*u)  SaturateOnIntegerOverflow=on  OutDataTypeStr=Inherit: Same as input  ParamDataTypeStr=Inherit: Same as input
  -a26 : Gain  Gain=-M1(2,3)-Ma1(2,3)  Multiplication=Matrix(K*u)  SaturateOnIntegerOverflow=on  OutDataTypeStr=Inherit: Same as input  ParamDataTypeStr=Inherit: Same as input
  Add : Sum
  Math Function : Math  Operator=magnitude^2  SignedPower=on  SaturateOnIntegerOverflow=on
  Product : Product  RndMeth=Zero
  x direction : Outport
  wires:
  v/1 -> Product/1
  r/1 -> Product/2, Math Function/1
  Product/1 -> -a22/1
  Math Function/1 -> -a26/1
  -a22/1 -> Add/1
  -a26/1 -> Add/2
  Add/1 -> x direction/1

== system Copy_of_towing_project1/local DP1/Tug/Coriolis and centripetal forces/Subsystem1 ==
  u : Inport
  r : Inport  Port=2
  Product : Product  RndMeth=Zero
  a11 : Gain  Gain=M1(1,1)+Ma1(1,1)  Multiplication=Matrix(K*u)  SaturateOnIntegerOverflow=on  OutDataTypeStr=Inherit: Same as input  ParamDataTypeStr=Inherit: Same as input
  y direction : Outport
  wires:
  Product/1 -> a11/1
  r/1 -> Product/2
  u/1 -> Product/1
  a11/1 -> y direction/1

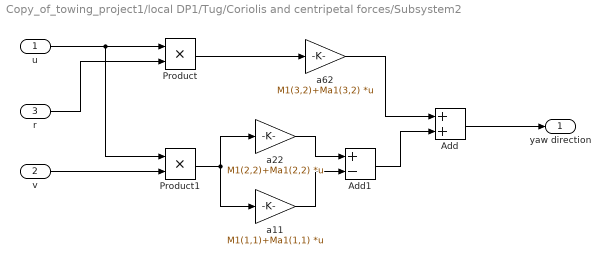
== system Copy_of_towing_project1/local DP1/Tug/Coriolis and centripetal forces/Subsystem2 ==
  u : Inport
  v : Inport  Port=2
  r : Inport  Port=3
  Add : Sum
  Add1 : Sum  Inputs=+-
  Product : Product  RndMeth=Zero
  Product1 : Product  RndMeth=Zero
  a11 : Gain  Gain=M1(1,1)+Ma1(1,1)  Multiplication=Matrix(K*u)  SaturateOnIntegerOverflow=on  OutDataTypeStr=Inherit: Same as input  ParamDataTypeStr=Inherit: Same as input
  a22 : Gain  Gain=M1(2,2)+Ma1(2,2)  Multiplication=Matrix(K*u)  SaturateOnIntegerOverflow=on  OutDataTypeStr=Inherit: Same as input  ParamDataTypeStr=Inherit: Same as input
  a62 : Gain  Gain=M1(3,2)+Ma1(3,2)  Multiplication=Matrix(K*u)  SaturateOnIntegerOverflow=on  OutDataTypeStr=Inherit: Same as input  ParamDataTypeStr=Inherit: Same as input
  yaw direction : Outport
  wires:
  u/1 -> Product/1, Product1/1
  r/1 -> Product/2
  Product/1 -> a62/1
  v/1 -> Product1/2
  Product1/1 -> a22/1, a11/1
  a22/1 -> Add1/1
  a11/1 -> Add1/2
  Add1/1 -> Add/2
  a62/1 -> Add/1
  Add/1 -> yaw direction/1

== matlab function MATLAB Function ==
  data: p0 input double; pd1 output double; v0 input double; state input double; pd2 output double
% function [pd1, pd2] = consensus_guidance(p0, v0, p1, v1, p2, v2)
function [pd1, pd2] = consensus_guidance(p0, v0, state)
% 默认输入和输出的单位为角度
% p(全局坐标系）， v(局部坐标系）
% dot_p (全局坐标系）
% clear all; clc;
% p1 = [397, 237, 31]';
% p2 = [397, -237, -31]';
% p0 = [1, 0, 0]';
% v0 = zeros(3, 1);
% v1 = zeros(3, 1);
% v2 = zeros(3, 1);
% p1 = state.getElement('state').Values(1).data
p1 = zeros(3, 1); v1 = p1;  p2 = p1;  v2 = p1;  
p1 = state(1:3);
v1 = state(4:6);
p2 = state(7:9);
v2 = state(10:12);

% 需要声明lqr函数为外部函数，否则simulink会编译报错
coder.extrinsic('lqr'); 

pd1 = zeros(3, 1);
pd2 = zeros(3, 1);

% 角度单位转化成弧度
deg_to_rad = pi / 180;
p0(3) = p0(3) * deg_to_rad;
p1(3) = p1(3) * deg_to_rad;
p2(3) = p2(3) * deg_to_rad;

dotP0 = V_to_dotP(p0, v0);
dotP1 = V_to_dotP(p1, v1);
dotP2 = V_to_dotP(p2, v2);
% 定义状态变量
x0 = [p0; dotP0];
x1 = [p1; dotP1];
x2 = [p2; dotP2];

%% 编队的相对位置
deta10 = [397, 237, 31 * deg_to_rad, 0, 0, 0]';
deta20 = [397, -237, -31 * deg_to_rad, 0, 0, 0]';
deta12 = [0, 474, 62 * deg_to_rad, 0, 0, 0]';
deta21 = -deta12;

% 先假定aij = 1, gi = 1;， 需要加上相对位置
e1 = x2 - x1 - deta21 + x0 - x1 + deta10;
e2 = x1 - x2 - deta12 + x0 - x2 + deta20;

%% 定义状态反馈方程的系数，求解raccati方程
wn = 0.05; 
cd = 0.7;

A1 = -2 * cd * wn * eye(3);
A0 = -wn^2 * eye(3);
B1 = -A0;

A = [zeros(3, 3), eye(3); A0, A1];
B = [zeros(3, 3); B1];

% Q = diag([0.01, 0.01, 4e-8, 100, 100, 4e-4]);
% R = diag([0.01, 0.01, 4e-8]);
Q = 4 * eye(6);
R = 1 * eye(3);
N = [];
[K, S, e] = lqr(A, B, Q, R, N);


u1 = K * e1;
u2 = K * e2;

pd1 = u1; 
pd2 = u2;

pd1 = pd1 + p1;
pd2 = pd2 + p2;

%% 函数输入输出都是角度
pd1(3) = pd1(3) / 3.14 * 180;
pd2(3) = pd2(3) / 3.14 * 180;

end







%% 旋转矩阵
function R = RotationMatrix(p)
fai = p(3);
R = zeros(3, 3);
R = [cos(fai), -sin(fai), 0;
    sin(fai), cos(fai), 0;
    0, 0, 1];
end

%% 将速度转换成全局坐标系中，即p的微分
function dot_P = V_to_dotP(p, v)
R = zeros(3, 3);
R = RotationMatrix(p);
dot_P = R * v;

end
